simulink model "EulerKinematics"  (R2021a)
settings: Solver=ode5  StartTime=0.0  StopTime=100  FixedStep=0.01  RelTol=1e-3
settings Model: Creator=PC  LastModifiedBy=PC

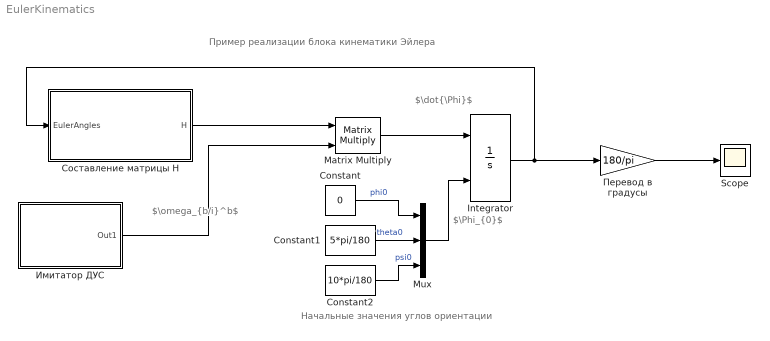
== system EulerKinematics ==
  note: Начальные значения углов ориентации
  note: $\dot{\Phi}$
  note: Пример реализации блока кинематики Эйлера
  note: $\omega_{b/i}^b$
  note: $\Phi_{0}$
  Constant : Constant  Value=0
  Constant1 : Constant  Value=5*pi/180
  Constant2 : Constant  Value=10*pi/180
  Integrator : Integrator  InitialConditionSource=external
  Matrix Multiply : Product  Multiplication=Matrix(*)
  Mux : Mux  Inputs=3
  Scope : Scope
  Имитатор ДУС : Subsystem
  Перевод в градусы : Gain  Gain=180/pi
  Составление матрицы H : MATLAB Function  TreatAsAtomicUnit=on
  wires:
  Составление матрицы H/1(H) -> Matrix Multiply/1
  Matrix Multiply/1 -> Integrator/1
  Имитатор ДУС/1(Out1) -> Matrix Multiply/2
  Integrator/1 -> Перевод в градусы/1, Составление матрицы H/1(EulerAngles)
  Mux/1 -> Integrator/2
  Constant/1 -> Mux/1  "phi0"
  Constant1/1 -> Mux/2  "theta0"
  Constant2/1 -> Mux/3  "psi0"
  Перевод в градусы/1 -> Scope/1

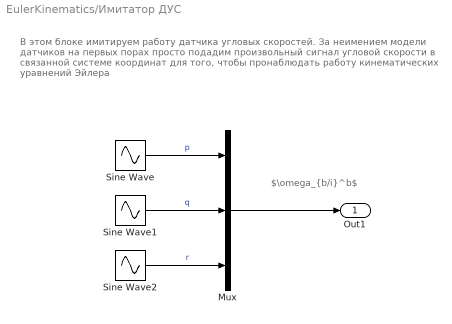
== system EulerKinematics/Имитатор ДУС ==
  note: $\omega_{b/i}^b$
  note: В этом блоке имитируем работу датчика угловых скоростей. За неимением модели датчиков на первых порах просто подадим произвольный сигнал угловой скорости в связанной системе координат для того, чтобы пронаблюдать работу кинематических уравнений Эйлера
  Mux : Mux  Inputs=3
  Sine Wave : Sin  Amplitude=10*pi/180 % амплитуда в радианах (10 градусов)  Frequency=5*pi/180  SampleTime=0
  Sine Wave1 : Sin  Amplitude=5*pi/180 % амплитуда в радианах (5 градусов)  Frequency=5*pi/180  SampleTime=0
  Sine Wave2 : Sin  Amplitude=1*pi/180 % амплитуда в радианах (5 градусов)  Frequency=5*pi/180  SampleTime=0
  Out1 : Outport
  wires:
  Mux/1 -> Out1/1
  Sine Wave/1 -> Mux/1  "p"
  Sine Wave1/1 -> Mux/2  "q"
  Sine Wave2/1 -> Mux/3  "r"

== matlab function EulerKinematics/Составление матрицы H ==
  data: EulerAngles input; H output
function H = fcn(EulerAngles)

% Извлекли из входного вектора углы ориентации
phi = EulerAngles(1);
theta = EulerAngles(2);
psi = EulerAngles(3); % Обратите внимание, что рыскание не нужно

% Составим матрицу системы кинематических уравнений Эйлера
H = [[1 tan(theta)*sin(phi) tan(theta)*cos(phi)];
    [0 cos(phi) -sin(phi)];
    [0 sin(phi)/cos(theta) cos(phi)/cos(theta)]];
